simulink model "BCM_C1A_EcuMonitor_4"  (Simulink 9.2)
settings: Solver=FixedStepDiscrete  StartTime=0.0  StopTime=5  FixedStep=0.01  RelTol=1e-3
undefined symbols (not defined in the file or in its folder): PRSK_DURATION_UNAVAILABLE_VALUE_CST, SECOND_TO_HUNDRED_MS_CST, TEN_CST, TYP_BCM_PRESOAK_REQUEST, TYP_HEVC_PRESOAK_ACTI_STATUS, TYP_LIN_LOW_LAYER, TYP_LOW_LAYER, TYP_RES_STATUS, TYP_UNDERHOOD_STATE, TYP_WAKE_UP_TYPE, ZERO_CST
libraries: Renault_Library x36, library_BCM x1
(part 2 of 2)

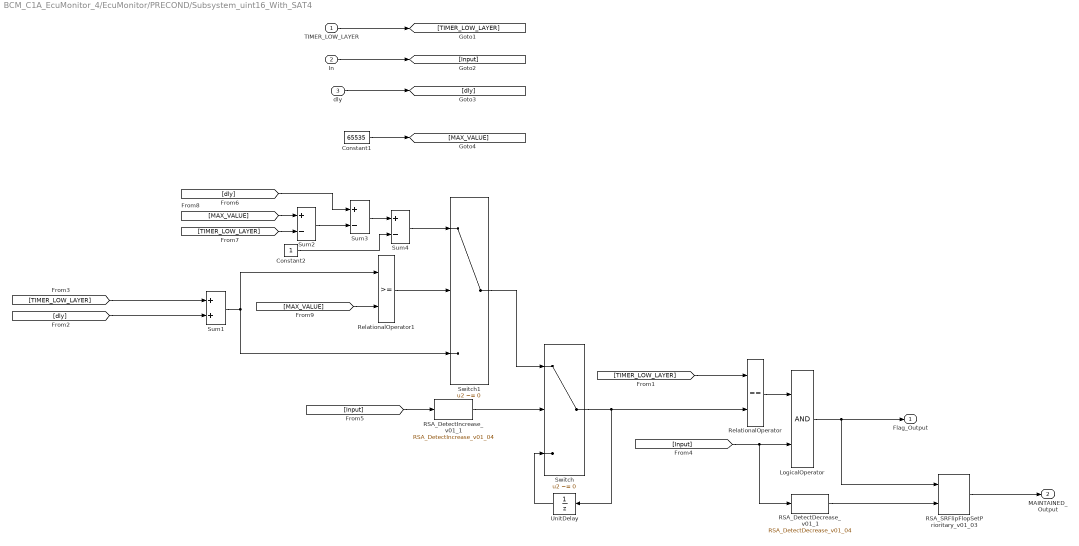
== system BCM_C1A_EcuMonitor_4/EcuMonitor/PRECOND/Subsystem_uint16_With_SAT4 ==
  TIMER_LOW_LAYER : Inport
      settings: AttributesFormatString=Type : %<OutDataTypeStr>
  In : Inport  Port=2
      settings: AttributesFormatString=Type : %<OutDataTypeStr>
  dly : Inport  Port=3
      settings: AttributesFormatString=Type : %<OutDataTypeStr>
  Constant1 : Constant  Value=65535  OutDataTypeStr=uint16  SampleTime=-1
  Constant2 : Constant  OutDataTypeStr=uint16  SampleTime=-1
  LogicalOperator : Logic  OutDataTypeStr=boolean
  RSA_DetectDecrease_v01_1 : Renault_Library/Complex blocks/Logic & Bit Operations/RSA_DetectDecrease_v01_04  Tag=[LIB]  chkini=on  vinit=0
      settings: AttributesFormatString=%<MaskType> : Ver : 01.04\nCompare the Input with Initial Value = %<chkini>\nInitial Value : = %<vinit>
  RSA_DetectIncrease_v01_1 : Renault_Library/Complex blocks/Logic & Bit Operations/RSA_DetectIncrease_v01_04  Tag=[LIB]  chkini=on  vinit=0
      settings: AttributesFormatString=%<MaskType> : Ver : 01.04\nCompare the Input with Initial Value = %<chkini>\nInitial Value : = %<vinit>
  RSA_SRFlipFlopSetPrioritary_v01_03 : Renault_Library/Complex blocks/Flip-Flop/RSA_SRFlipFlopSetPrioritary_v01_03  Tag=[LIB]  init=false
      settings: AttributesFormatString=%<MaskType> : Ver : 01.03\n<init=%<init>>
  RelationalOperator : RelationalOperator  Operator===  OutDataTypeStr=boolean  RndMeth=Nearest  InputSameDT=on
  RelationalOperator1 : RelationalOperator  OutDataTypeStr=boolean  RndMeth=Nearest  InputSameDT=on
  Sum1 : Sum  AccumDataTypeStr=uint16  OutDataTypeStr=Inherit: Inherit via back propagation  RndMeth=Zero  SaturateOnIntegerOverflow=on  InputSameDT=on
  Sum2 : Sum  Inputs=+-  AccumDataTypeStr=uint16  OutDataTypeStr=Inherit: Inherit via back propagation  RndMeth=Zero  SaturateOnIntegerOverflow=on  InputSameDT=on
  Sum3 : Sum  Inputs=+-  AccumDataTypeStr=uint16  OutDataTypeStr=Inherit: Inherit via back propagation  RndMeth=Zero  SaturateOnIntegerOverflow=on  InputSameDT=on
  Sum4 : Sum  Inputs=+-  AccumDataTypeStr=uint16  OutDataTypeStr=Inherit: Inherit via back propagation  RndMeth=Zero  SaturateOnIntegerOverflow=on  InputSameDT=on
  Switch : Switch  Criteria=u2 ~= 0  RndMeth=Zero  InputSameDT=on
      settings: AttributesFormatString=Criteria=%<Criteria>
  Switch1 : Switch  Criteria=u2 ~= 0  RndMeth=Zero  InputSameDT=on
      settings: AttributesFormatString=Criteria=%<Criteria>
  UnitDelay : UnitDelay  SampleTime=-1
      settings: AttributesFormatString=IC = %<X0>
  Flag_Output : Outport
      settings: AttributesFormatString=Type : %<OutDataTypeStr>\nInit :%<InitialOutput>
  MAINTAINED_Output : Outport  Port=2
      settings: AttributesFormatString=Type : %<OutDataTypeStr>\nInit :%<InitialOutput>
  wires:
  Switch1/1 -> Switch/1
  Sum4/1 -> Switch1/1
  Constant2/1 -> Sum4/2
  Sum3/1 -> Sum4/1
  Sum2/1 -> Sum3/2
  [dly] -> Sum3/1
  [TIMER_LOW_LAYER] -> Sum2/2
  [dly] -> Sum1/2
  dly/1 -> [dly]
  RelationalOperator1/1 -> Switch1/2
  Switch/1 -> UnitDelay/1, RelationalOperator/2
  Sum1/1 -> RelationalOperator1/1, Switch1/3
  LogicalOperator/1 -> RSA_SRFlipFlopSetPrioritary_v01_03/1, Flag_Output/1
  RSA_DetectIncrease_v01_1/1 -> Switch/2
  [Input] -> RSA_DetectIncrease_v01_1/1
  In/1 -> [Input]
  TIMER_LOW_LAYER/1 -> [TIMER_LOW_LAYER]
  [TIMER_LOW_LAYER] -> Sum1/1
  UnitDelay/1 -> Switch/3
  [TIMER_LOW_LAYER] -> RelationalOperator/1
  [Input] -> RSA_DetectDecrease_v01_1/1, LogicalOperator/2
  RelationalOperator/1 -> LogicalOperator/1
  RSA_DetectDecrease_v01_1/1 -> RSA_SRFlipFlopSetPrioritary_v01_03/2
  RSA_SRFlipFlopSetPrioritary_v01_03/1 -> MAINTAINED_Output/1
  Constant1/1 -> [MAX_VALUE]
  [MAX_VALUE] -> Sum2/1
  [MAX_VALUE] -> RelationalOperator1/2

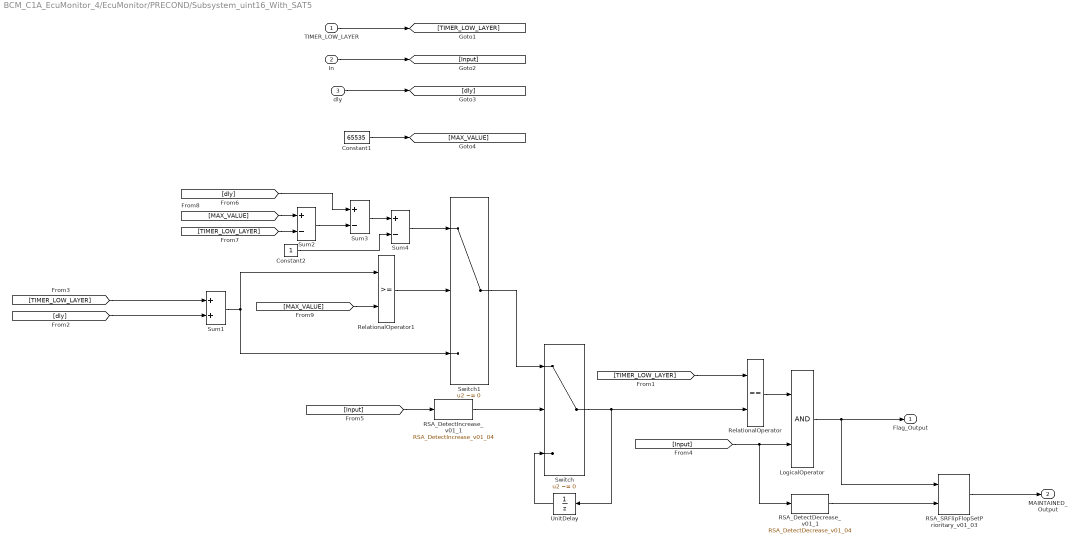
== system BCM_C1A_EcuMonitor_4/EcuMonitor/PRECOND/Subsystem_uint16_With_SAT5 ==
  TIMER_LOW_LAYER : Inport
      settings: AttributesFormatString=Type : %<OutDataTypeStr>
  In : Inport  Port=2
      settings: AttributesFormatString=Type : %<OutDataTypeStr>
  dly : Inport  Port=3
      settings: AttributesFormatString=Type : %<OutDataTypeStr>
  Constant1 : Constant  Value=65535  OutDataTypeStr=uint16  SampleTime=-1
  Constant2 : Constant  OutDataTypeStr=uint16  SampleTime=-1
  LogicalOperator : Logic  OutDataTypeStr=boolean
  RSA_DetectDecrease_v01_1 : Renault_Library/Complex blocks/Logic & Bit Operations/RSA_DetectDecrease_v01_04  Tag=[LIB]  chkini=on  vinit=0
      settings: AttributesFormatString=%<MaskType> : Ver : 01.04\nCompare the Input with Initial Value = %<chkini>\nInitial Value : = %<vinit>
  RSA_DetectIncrease_v01_1 : Renault_Library/Complex blocks/Logic & Bit Operations/RSA_DetectIncrease_v01_04  Tag=[LIB]  chkini=on  vinit=0
      settings: AttributesFormatString=%<MaskType> : Ver : 01.04\nCompare the Input with Initial Value = %<chkini>\nInitial Value : = %<vinit>
  RSA_SRFlipFlopSetPrioritary_v01_03 : Renault_Library/Complex blocks/Flip-Flop/RSA_SRFlipFlopSetPrioritary_v01_03  Tag=[LIB]  init=false
      settings: AttributesFormatString=%<MaskType> : Ver : 01.03\n<init=%<init>>
  RelationalOperator : RelationalOperator  Operator===  OutDataTypeStr=boolean  RndMeth=Nearest  InputSameDT=on
  RelationalOperator1 : RelationalOperator  OutDataTypeStr=boolean  RndMeth=Nearest  InputSameDT=on
  Sum1 : Sum  AccumDataTypeStr=uint16  OutDataTypeStr=Inherit: Inherit via back propagation  RndMeth=Zero  SaturateOnIntegerOverflow=on  InputSameDT=on
  Sum2 : Sum  Inputs=+-  AccumDataTypeStr=uint16  OutDataTypeStr=Inherit: Inherit via back propagation  RndMeth=Zero  SaturateOnIntegerOverflow=on  InputSameDT=on
  Sum3 : Sum  Inputs=+-  AccumDataTypeStr=uint16  OutDataTypeStr=Inherit: Inherit via back propagation  RndMeth=Zero  SaturateOnIntegerOverflow=on  InputSameDT=on
  Sum4 : Sum  Inputs=+-  AccumDataTypeStr=uint16  OutDataTypeStr=Inherit: Inherit via back propagation  RndMeth=Zero  SaturateOnIntegerOverflow=on  InputSameDT=on
  Switch : Switch  Criteria=u2 ~= 0  RndMeth=Zero  InputSameDT=on
      settings: AttributesFormatString=Criteria=%<Criteria>
  Switch1 : Switch  Criteria=u2 ~= 0  RndMeth=Zero  InputSameDT=on
      settings: AttributesFormatString=Criteria=%<Criteria>
  UnitDelay : UnitDelay  SampleTime=-1
      settings: AttributesFormatString=IC = %<X0>
  Flag_Output : Outport
      settings: AttributesFormatString=Type : %<OutDataTypeStr>\nInit :%<InitialOutput>
  MAINTAINED_Output : Outport  Port=2
      settings: AttributesFormatString=Type : %<OutDataTypeStr>\nInit :%<InitialOutput>
  wires:
  Switch1/1 -> Switch/1
  Sum4/1 -> Switch1/1
  Constant2/1 -> Sum4/2
  Sum3/1 -> Sum4/1
  Sum2/1 -> Sum3/2
  [dly] -> Sum3/1
  [TIMER_LOW_LAYER] -> Sum2/2
  [dly] -> Sum1/2
  dly/1 -> [dly]
  RelationalOperator1/1 -> Switch1/2
  Switch/1 -> UnitDelay/1, RelationalOperator/2
  Sum1/1 -> RelationalOperator1/1, Switch1/3
  LogicalOperator/1 -> RSA_SRFlipFlopSetPrioritary_v01_03/1, Flag_Output/1
  RSA_DetectIncrease_v01_1/1 -> Switch/2
  [Input] -> RSA_DetectIncrease_v01_1/1
  In/1 -> [Input]
  TIMER_LOW_LAYER/1 -> [TIMER_LOW_LAYER]
  [TIMER_LOW_LAYER] -> Sum1/1
  UnitDelay/1 -> Switch/3
  [TIMER_LOW_LAYER] -> RelationalOperator/1
  [Input] -> RSA_DetectDecrease_v01_1/1, LogicalOperator/2
  RelationalOperator/1 -> LogicalOperator/1
  RSA_DetectDecrease_v01_1/1 -> RSA_SRFlipFlopSetPrioritary_v01_03/2
  RSA_SRFlipFlopSetPrioritary_v01_03/1 -> MAINTAINED_Output/1
  Constant1/1 -> [MAX_VALUE]
  [MAX_VALUE] -> Sum2/1
  [MAX_VALUE] -> RelationalOperator1/2

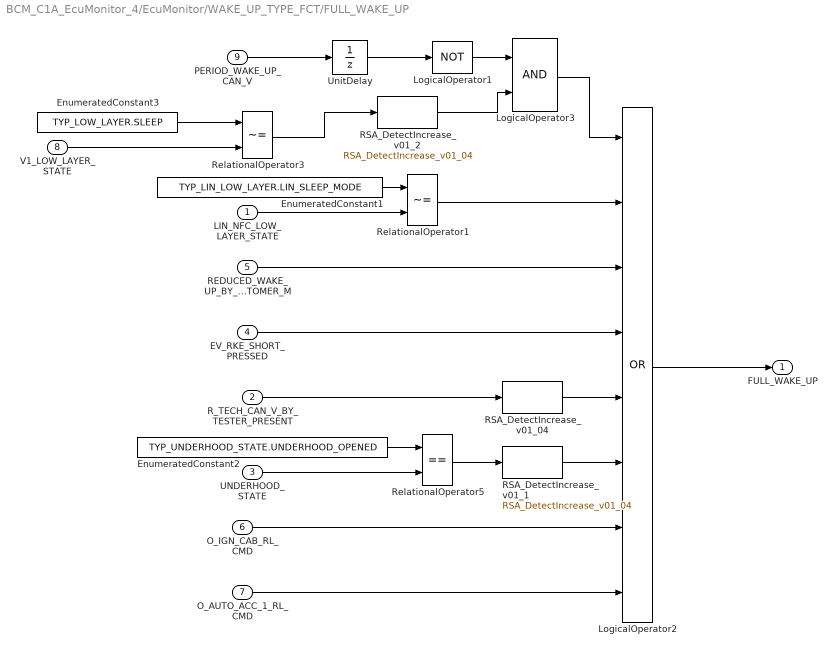
== system BCM_C1A_EcuMonitor_4/EcuMonitor/WAKE_UP_TYPE_FCT/FULL_WAKE_UP ==
  LIN_NFC_LOW_LAYER_STATE : Inport
      settings: AttributesFormatString=Type : %<OutDataTypeStr>
  R_TECH_CAN_V_BY_TESTER_PRESENT : Inport  Port=2
      settings: AttributesFormatString=Type : %<OutDataTypeStr>
  UNDERHOOD_STATE : Inport  Port=3
      settings: AttributesFormatString=Type : %<OutDataTypeStr>
  EV_RKE_SHORT_PRESSED : Inport  Port=4
      settings: AttributesFormatString=Type : %<OutDataTypeStr>
  REDUCED_WAKE_UP_BY_CUSTOMER_M : Inport  Port=5
      settings: AttributesFormatString=Type : %<OutDataTypeStr>
  O_IGN_CAB_RL_CMD : Inport  Port=6
  O_AUTO_ACC_1_RL_CMD : Inport  Port=7
  V1_LOW_LAYER_STATE : Inport  Port=8
      settings: AttributesFormatString=Type : %<OutDataTypeStr>
  PERIOD_WAKE_UP_CAN_V : Inport  Port=9
      settings: AttributesFormatString=Type : %<OutDataTypeStr>
  EnumeratedConstant1 : Constant  Value=TYP_LIN_LOW_LAYER.LIN_SLEEP_MODE  OutDataTypeStr=Enum: TYP_LIN_LOW_LAYER  SampleTime=-1
  EnumeratedConstant2 : Constant  Value=TYP_UNDERHOOD_STATE.UNDERHOOD_OPENED  OutDataTypeStr=Enum: TYP_UNDERHOOD_STATE  SampleTime=-1
  EnumeratedConstant3 : Constant  Value=TYP_LOW_LAYER.SLEEP  OutDataTypeStr=Enum: TYP_LOW_LAYER  SampleTime=-1
  LogicalOperator1 : Logic  Operator=NOT  Inputs=8  OutDataTypeStr=boolean
  LogicalOperator2 : Logic  Operator=OR  Inputs=8  OutDataTypeStr=boolean
  LogicalOperator3 : Logic  OutDataTypeStr=boolean
  RSA_DetectIncrease_v01_04 : Renault_Library/Complex blocks/Logic & Bit Operations/RSA_DetectIncrease_v01_04  Tag=[LIB]  chkini=on  vinit=0
      settings: AttributesFormatString=%<MaskType> : Ver : 01.04\nCompare the Input with Initial Value = %<chkini>\nInitial Value : = %<vinit>
  RSA_DetectIncrease_v01_1 : Renault_Library/Complex blocks/Logic & Bit Operations/RSA_DetectIncrease_v01_04  Tag=[LIB]  chkini=on  vinit=0
      settings: AttributesFormatString=%<MaskType> : Ver : 01.04\nCompare the Input with Initial Value = %<chkini>\nInitial Value : = %<vinit>
  RSA_DetectIncrease_v01_2 : Renault_Library/Complex blocks/Logic & Bit Operations/RSA_DetectIncrease_v01_04  Tag=[LIB]  chkini=on  vinit=0
      settings: AttributesFormatString=%<MaskType> : Ver : 01.04\nCompare the Input with Initial Value = %<chkini>\nInitial Value : = %<vinit>
  RelationalOperator1 : RelationalOperator  Operator=~=  OutDataTypeStr=boolean  RndMeth=Nearest  InputSameDT=on
  RelationalOperator3 : RelationalOperator  Operator=~=  OutDataTypeStr=boolean  RndMeth=Nearest  InputSameDT=on
  RelationalOperator5 : RelationalOperator  Operator===  OutDataTypeStr=boolean  RndMeth=Nearest  InputSameDT=on
  UnitDelay : UnitDelay  SampleTime=-1
      settings: AttributesFormatString=IC = %<X0>
  FULL_WAKE_UP : Outport
      settings: AttributesFormatString=Type : %<OutDataTypeStr>\nInit :%<InitialOutput>
  wires:
  LogicalOperator2/1 -> FULL_WAKE_UP/1
  R_TECH_CAN_V_BY_TESTER_PRESENT/1 -> RSA_DetectIncrease_v01_04/1
  UNDERHOOD_STATE/1 -> RelationalOperator5/2
  EnumeratedConstant2/1 -> RelationalOperator5/1
  LIN_NFC_LOW_LAYER_STATE/1 -> RelationalOperator1/2
  RelationalOperator5/1 -> RSA_DetectIncrease_v01_1/1
  EnumeratedConstant1/1 -> RelationalOperator1/1
  O_IGN_CAB_RL_CMD/1 -> LogicalOperator2/7
  O_AUTO_ACC_1_RL_CMD/1 -> LogicalOperator2/8
  V1_LOW_LAYER_STATE/1 -> RelationalOperator3/2
  EnumeratedConstant3/1 -> RelationalOperator3/1
  RSA_DetectIncrease_v01_04/1 -> LogicalOperator2/5
  RSA_DetectIncrease_v01_1/1 -> LogicalOperator2/6
  EV_RKE_SHORT_PRESSED/1 -> LogicalOperator2/4
  REDUCED_WAKE_UP_BY_CUSTOMER_M/1 -> LogicalOperator2/3
  RelationalOperator1/1 -> LogicalOperator2/2
  RelationalOperator3/1 -> RSA_DetectIncrease_v01_2/1
  PERIOD_WAKE_UP_CAN_V/1 -> UnitDelay/1
  LogicalOperator1/1 -> LogicalOperator3/1
  LogicalOperator3/1 -> LogicalOperator2/1
  RSA_DetectIncrease_v01_2/1 -> LogicalOperator3/2
  UnitDelay/1 -> LogicalOperator1/1

== system BCM_C1A_EcuMonitor_4/EcuMonitor/WAKE_UP_TYPE_FCT/SELECTIVE_MODE ==
  PERIOD_WAKE_UP_CAN_V : Inport
      settings: AttributesFormatString=Type : %<OutDataTypeStr>
  BCM_MONITOR_REFUSE_TO_SLEEP : Inport  Port=2
      settings: AttributesFormatString=Type : %<OutDataTypeStr>
  LogicalOperator6 : Logic  Operator=OR  OutDataTypeStr=boolean
  RSA_DetectDecrease_v01_04 : Renault_Library/Complex blocks/Logic & Bit Operations/RSA_DetectDecrease_v01_04  Tag=[LIB]  chkini=on  vinit=0
      settings: AttributesFormatString=%<MaskType> : Ver : 01.04\nCompare the Input with Initial Value = %<chkini>\nInitial Value : = %<vinit>
  RSA_DetectIncrease_v01_04 : Renault_Library/Complex blocks/Logic & Bit Operations/RSA_DetectIncrease_v01_04  Tag=[LIB]  chkini=on  vinit=0
      settings: AttributesFormatString=%<MaskType> : Ver : 01.04\nCompare the Input with Initial Value = %<chkini>\nInitial Value : = %<vinit>
  SELECTIVE_MODE : Outport
      settings: AttributesFormatString=Type : %<OutDataTypeStr>\nInit :%<InitialOutput>
  wires:
  LogicalOperator6/1 -> SELECTIVE_MODE/1
  PERIOD_WAKE_UP_CAN_V/1 -> RSA_DetectIncrease_v01_04/1
  BCM_MONITOR_REFUSE_TO_SLEEP/1 -> RSA_DetectDecrease_v01_04/1
  RSA_DetectIncrease_v01_04/1 -> LogicalOperator6/2
  RSA_DetectDecrease_v01_04/1 -> LogicalOperator6/1

== system BCM_C1A_EcuMonitor_4/EcuMonitor/WAKE_UP_TYPE_FCT/WAKE_UP_TYPE_SELECTION ==
  FULL_WAKE_UP : Inport
      settings: AttributesFormatString=Type : %<OutDataTypeStr>
  SELECTIVE_MODE : Inport  Port=2
      settings: AttributesFormatString=Type : %<OutDataTypeStr>
  EnumeratedConstant1 : Constant  Value=TYP_WAKE_UP_TYPE.SELECTIVE_WAKE_UP_MODE_1  OutDataTypeStr=Enum: TYP_WAKE_UP_TYPE  SampleTime=-1
  EnumeratedConstant2 : Constant  Value=TYP_WAKE_UP_TYPE.FULL_WAKE_UP  OutDataTypeStr=Enum: TYP_WAKE_UP_TYPE  SampleTime=-1
  RSA_SRFlipFlopSetPrioritary_v01_03 : Renault_Library/Complex blocks/Flip-Flop/RSA_SRFlipFlopSetPrioritary_v01_03  Tag=[LIB]  init=false
      settings: AttributesFormatString=%<MaskType> : Ver : 01.03\n<init=%<init>>
  Switch : Switch  Criteria=u2 ~= 0  RndMeth=Zero  InputSameDT=on
      settings: AttributesFormatString=Criteria=%<Criteria>
  WAKE_UP_TYPE : Outport
      settings: AttributesFormatString=Type : %<OutDataTypeStr>\nInit :%<InitialOutput>
  wires:
  SELECTIVE_MODE/1 -> RSA_SRFlipFlopSetPrioritary_v01_03/2
  FULL_WAKE_UP/1 -> RSA_SRFlipFlopSetPrioritary_v01_03/1
  Switch/1 -> WAKE_UP_TYPE/1
  EnumeratedConstant2/1 -> Switch/1
  EnumeratedConstant1/1 -> Switch/3
  RSA_SRFlipFlopSetPrioritary_v01_03/1 -> Switch/2
